simulink model "frontal"  (R2019b)
settings: Solver=VariableStepAuto  StartTime=0.0  StopTime=5  RelTol=1e-3
undefined symbols (not defined in the file): Kx, x0, xr
settings Model: Creator=mmaximo  LastModifiedBy=rodri

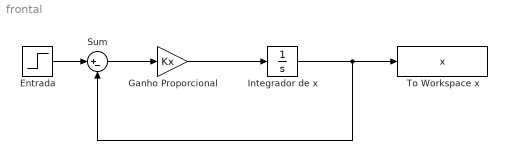
== system frontal ==
  Entrada : Step  Time=0  Before=x0  After=xr  SampleTime=0
  Ganho Proporcional : Gain  Gain=Kx
  Integrador de x : Integrator
  Sum : Sum  Inputs=|+-
  To Workspace x : ToWorkspace  VariableName=x  SaveFormat=Structure With Time  SampleTime=-1
  wires:
  Sum/1 -> Ganho Proporcional/1
  Entrada/1 -> Sum/1
  Ganho Proporcional/1 -> Integrador de x/1
  Integrador de x/1 -> Sum/2, To Workspace x/1
